simulink model "module_dynamic_merge_2018b"  (R2018b)
settings: Solver=FixedStepAuto  StartTime=0.0  StopTime=inf  FixedStep=0.001  RelTol=1e-3
settings Model: DataDictionary=LCplanning.sldd  Creator=lenovo  LastModifiedBy=lenovo
settings DataIOCC: ReturnWorkspaceOutputs=on

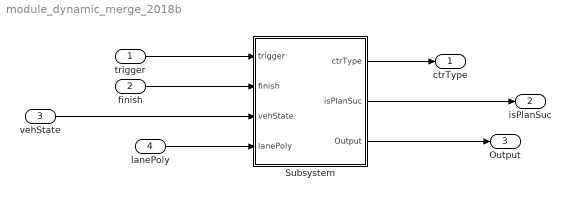
== system module_dynamic_merge_2018b ==
  trigger : Inport
  finish : Inport  Port=2
  vehState : Inport  Port=3  OutDataTypeStr=Bus: vehStates
  "lanePoly " : Inport  Port=4  OutDataTypeStr=Bus: lanePoly
  Subsystem : Subsystem
  ctrType : Outport  OutDataTypeStr=double
  isPlanSuc : Outport  Port=2  OutDataTypeStr=int8
  Output : Outport  Port=3  OutDataTypeStr=Bus: PlanningOutput
  wires:
  trigger/1 -> Subsystem/1(trigger)
  finish/1 -> Subsystem/2(finish)
  vehState/1 -> Subsystem/3(vehState)
  "lanePoly "/1 -> Subsystem/4("lanePoly ")
  Subsystem/1(ctrType) -> ctrType/1
  Subsystem/2(isPlanSuc) -> isPlanSuc/1
  Subsystem/3(Output) -> Output/1

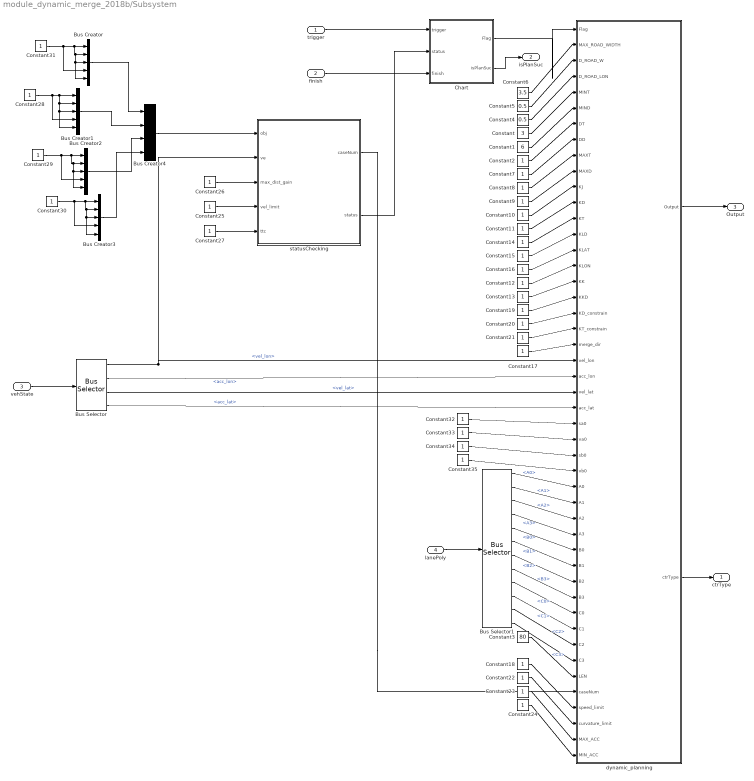
== system module_dynamic_merge_2018b/Subsystem ==
  trigger : Inport
  finish : Inport  Port=2
  vehState : Inport  Port=3  OutDataTypeStr=Bus: vehStates
  "lanePoly " : Inport  Port=4  OutDataTypeStr=Bus: lanePoly
  Bus Creator{,1..3} (4 alike) : BusCreator  Inputs=5  OutDataTypeStr=Bus: ObjInfo
  Bus Creator4 : BusCreator  Inputs=4  OutDataTypeStr=Bus: SelectedObject
  Bus Selector : BusSelector  OutputSignals=vel_lon,acc_lon,vel_lat,acc_lat
  Bus Selector1 : BusSelector  OutputSignals=A0,A1,A2,A3,B0,B1,B2,B3,C0,C1,C2,C3
  Chart : Stateflow chart  TreatAsAtomicUnit=on
  Constant : Constant  Value=3
  Constant1 : Constant  Value=6
  Constant{2,7..35} (30 alike) : Constant
  Constant3 : Constant  Value=80  OutDataTypeStr=double
  Constant4 : Constant  Value=0.5
  Constant5 : Constant  Value=0.5
  Constant6 : Constant  Value=3.5
  dynamic_planning : MATLAB Function  TreatAsAtomicUnit=on
  statusChecking : MATLAB Function  TreatAsAtomicUnit=on
  ctrType : Outport  OutDataTypeStr=double
  isPlanSuc : Outport  Port=2  OutDataTypeStr=int8
  Output : Outport  Port=3  OutDataTypeStr=Bus: PlanningOutput
  wires:
  Constant2/1 -> dynamic_planning/7(DT)
  Constant5/1 -> dynamic_planning/3(D_ROAD_W)
  Bus Selector1/10 -> dynamic_planning/39(C1)  "<C1>"
  Constant19/1 -> dynamic_planning/18(KKD)
  Bus Creator4/1 -> statusChecking/1(obj)
  trigger/1 -> Chart/1(trigger)
  Constant/1 -> dynamic_planning/5(MINT)
  statusChecking/1(caseNum) -> dynamic_planning/43(caseNum)
  Bus Selector1/5 -> dynamic_planning/34(B0)  "<B0>"
  statusChecking/2(status) -> Chart/2(status)
  Constant11/1 -> dynamic_planning/12(KD)
  Constant34/1 -> dynamic_planning/28(sb0)
  Constant14/1 -> dynamic_planning/13(KT)
  Constant10/1 -> dynamic_planning/11(KJ)
  Chart/1(Flag) -> dynamic_planning/1(Flag)
  Bus Creator/1 -> Bus Creator4/1
  Bus Creator3/1 -> Bus Creator4/4
  Constant4/1 -> dynamic_planning/4(D_ROAD_LON)
  Constant27/1 -> statusChecking/5(ttc)
  Constant15/1 -> dynamic_planning/14(KLD)
  Constant33/1 -> dynamic_planning/27(va0)
  "lanePoly "/1 -> Bus Selector1/1
  Bus Selector/3 -> dynamic_planning/24(vel_lat)  "<vel_lat>"
  Bus Selector1/2 -> dynamic_planning/31(A1)  "<A1>"
  Bus Selector1/7 -> dynamic_planning/36(B2)  "<B2>"
  Constant16/1 -> dynamic_planning/15(KLAT)
  Constant1/1 -> dynamic_planning/6(MIND)
  Bus Creator2/1 -> Bus Creator4/3
  Constant17/1 -> dynamic_planning/21(merge_dir)
  finish/1 -> Chart/3(finish)
  Bus Selector1/12 -> dynamic_planning/41(C3)  "<C3>"
  Constant13/1 -> dynamic_planning/17(KK)
  Constant3/1 -> dynamic_planning/42(LEN)
  Constant30/1 -> Bus Creator3/4, Bus Creator3/3, Bus Creator3/5, Bus Creator3/2, Bus Creator3/1
  Constant31/1 -> Bus Creator/4, Bus Creator/3, Bus Creator/5, Bus Creator/2, Bus Creator/1
  Constant12/1 -> dynamic_planning/16(KLON)
  Bus Selector1/11 -> dynamic_planning/40(C2)  "<C2>"
  Bus Selector/1 -> statusChecking/2(ve), dynamic_planning/22(vel_lon)  "<vel_lon>"
  Constant20/1 -> dynamic_planning/19(KD_constrain)
  Bus Selector/4 -> dynamic_planning/25(acc_lat)  "<acc_lat>"
  Constant6/1 -> dynamic_planning/2(MAX_ROAD_WIDTH)
  dynamic_planning/2(ctrType) -> ctrType/1
  Chart/2(isPlanSuc) -> isPlanSuc/1
  Constant9/1 -> dynamic_planning/10(MAXD)
  Constant29/1 -> Bus Creator2/4, Bus Creator2/3, Bus Creator2/5, Bus Creator2/2, Bus Creator2/1
  vehState/1 -> Bus Selector/1
  Bus Selector1/9 -> dynamic_planning/38(C0)  "<C0>"
  dynamic_planning/1(Output) -> Output/1
  Constant22/1 -> dynamic_planning/45(curvature_limit)
  Constant28/1 -> Bus Creator1/4, Bus Creator1/1, Bus Creator1/2, Bus Creator1/3, Bus Creator1/5
  Constant7/1 -> dynamic_planning/8(DD)
  Constant25/1 -> statusChecking/4(vel_limit)
  Constant23/1 -> dynamic_planning/46(MAX_ACC)
  Constant24/1 -> dynamic_planning/47(MIN_ACC)
  Constant26/1 -> statusChecking/3(max_dist_gain)
  Bus Selector1/4 -> dynamic_planning/33(A3)  "<A3>"
  Constant21/1 -> dynamic_planning/20(KT_constrain)
  Constant8/1 -> dynamic_planning/9(MAXT)
  Bus Selector/2 -> dynamic_planning/23(acc_lon)  "<acc_lon>"
  Bus Creator1/1 -> Bus Creator4/2
  Bus Selector1/1 -> dynamic_planning/30(A0)  "<A0>"
  Constant35/1 -> dynamic_planning/29(vb0)
  Constant18/1 -> dynamic_planning/44(speed_limit)
  Bus Selector1/8 -> dynamic_planning/37(B3)  "<B3>"
  Bus Selector1/3 -> dynamic_planning/32(A2)  "<A2>"
  Bus Selector1/6 -> dynamic_planning/35(B1)  "<B1>"
  Constant32/1 -> dynamic_planning/26(sa0)

== matlab function module_dynamic_merge_2018b/Subsystem/dynamic_planning ==
  data: Flag input; MAX_ROAD_WIDTH input; Output output Bus: PlanningOutput; D_ROAD_W input; D_ROAD_LON input; MINT input; MIND input; DT input; DD input; MAXT input; MAXD input; KJ input; KD input; KT input; KLD input; KLAT input; KLON input; KK input; KKD input; KD_constrain input; KT_constrain input; merge_dir input; vel_lon input; acc_lon input; vel_lat input; acc_lat input; sa0 input; va0 input; sb0 input; vb0 input; A0 input; A1 input; A2 input; A3 input; B0 input; B1 input; B2 input; B3 input; C0 input; C1 input; C2 input; C3 input; LEN input; caseNum input; speed_limit input; curvature_limit input; MAX_ACC input; MIN_ACC input; ctrType output double
%% /****************************************************************************
% *  Automatic Lane Changing                                                   *
% *  Copyright (C) 2020 Yuncheng JIANG  yjiangbw@connect.ust.hk.               *
% *                                                                            *
% *  This file is part of Lane Changing functionals.                           *
% *                                                                            *
% *  This program is free software; you can redistribute it and/or modify      *
% *  it under the terms of the GNU General Public License version 3 as         *
% *  published by the Free Software Foundation.                                *
% *                                                                            *
% *  You should have received a copy of the GNU General Public License         *
% *  along with OST. If not, see <http://www.gnu.org/licenses/>.               *
% *                                                                            *
% *  Unless required by applicable law or agreed to in writing, software       *
% *  distributed under the License is distributed on an "AS IS" BASIS,         *
% *  WITHOUT WARRANTIES OR CONDITIONS OF ANY KIND, either express or implied.  *
% *  See the License for the specific language governing permissions and       *
% *  limitations under the License.                                            *
% *                                                                            *
% *  @file                                                                     *
% *  @brief                                                                    *
% *  Details.                                                                  *
% *                                                                            *
% *  @author   Yuncheng.JIANG                                                  *
% *  @email    yjiangbw@connect.ust.hk.                                        *
% *  @version  1.0.0.1( )                                                      *
% *  @date     /12/1/2020                                                      *
% *  @license  GNU General Public License (GPL)                                *
% *                                                                            *
% *----------------------------------------------------------------------------*
% *  Remark         : Description                                              *
% *----------------------------------------------------------------------------*
% *  Change History :                                                          *
% *  <Date>     | <Version> | <Author>       | <Description>                   *
% *----------------------------------------------------------------------------*
% *  2020/12/01 | 1.0.0.1   | Yuncheng.JIANG       | Create file               *
% *----------------------------------------------------------------------------*
% *                                                                            *
% *****************************************************************************/

%% following is the parameter value reference

% global MAX_ROAD_WIDTH D_ROAD_W D_ROAD_LON MINT MIND DT DD MAXT MAXD KJ KD KT KLD KLAT KLON KK KKD KD_constrain KT_constrain;
% global merge_dir lat_offset vel_lon acc_lon vel_lat acc_lat ; 
% global sa0 va0 sb0 vb0 
% global A0 A1 A2 A3 B0 B1 B2 B3
% global LEN caseNum
% global speed_limit curvature_limit MAX_ACC MIN_ACC
% 
% MAX_ROAD_WIDTH = 3 ; %  [m]
% D_ROAD_W = 0.5 ; %  [m]
% D_ROAD_LON = 0.5;
% DT = 1 ; % Delta T [s]
% MAXT = 6;% [s]
% MINT = 3; % [s]
% DD = 1 ; % Delta T [s]
% MAXD = 80;% [s]
% MIND = 40; % [s]
% KJ = 0.1;
% KT = 0.1;
% KD = 1;
% KLD = 1;
% KLAT = 1;
% KLON = 1;
% KK = 1;
% KKD = 1;
% KD_constrain = 0.1;
% KT_constrain = 1;
% 
% merge_dir = 1;
% vel_lon = 10;
% acc_lon = 0;
% vel_lat = 0;
% acc_lat = 0;
% lat_offset = -6;
% 
% sa0 = 0;
% va0 = 10;
% sb0 = 15;
% vb0 = 10; 
% 
% A0 = -3; A1 = -0.1; A2 = -0.001; A3 = -0.0001;
% B0 = 3; B1 = -0.1; B2 = -0.001; B3 = -0.00008;
% % we also have C parameters here
% 
% LEN = 80;
% caseNum = 2;
% speed_limit = 33.3; % which is 120kph;
% curvature_limit = 1/50;
% MAX_ACC = 4;
% MIN_ACC = -4;


%% the test declare that when caseNum == 4, it is a free lane changing.
% when caseNum != 4, it is merging lane changing.


%%
% frenet_data = check_status(cost_graph);
% cost_total = frenet_data(1);
% Te = frenet_data(2);
% de = frenet_data(3);
% se = frenet_data(4);
% [y_of_x,p_of_v,p_of_a] = conbination(frenet_data);
% toc; 
% 
% fprintf("the calculation time = %f  ms \r",1000*toc);
% 
% figure
% plot(p_of_v(:,1),p_of_v(:,2));
% title("y of x");
% figure
% plot(p_of_v(:,1),p_of_v(:,3));
% title("p of v");
% figure
% plot(p_of_a(:,1),p_of_a(:,3));
% title("p of a");

%%
function [Output,ctrType]  = dynamic_planning(Flag, MAX_ROAD_WIDTH, D_ROAD_W, D_ROAD_LON,...
    MINT, MIND, DT, DD, MAXT, MAXD, KJ, KD, KT, KLD, KLAT, KLON, KK, KKD, KD_constrain, KT_constrain,...
    merge_dir, vel_lon, acc_lon, vel_lat, acc_lat,...
    sa0, va0, sb0, vb0 ,A0, A1, A2, A3, B0, B1, B2, B3, C0, C1, C2, C3,LEN, caseNum,...
    speed_limit, curvature_limit, MAX_ACC, MIN_ACC)
    %% this function discrriminate two different sampling methods.
    % if caseNum ==4, it means this is simple lane changing, we change lane
    % without considering of velocity planning
    % if caseNum != 4, it means this is merging lane changing, we apply
    % x(t)-y(t) method to plan spatially and temporally. 
    
%     global Flag MAX_ROAD_WIDTH D_ROAD_W D_ROAD_LON MINT MIND DT DD MAXT MAXD KJ KD KT KLD KLAT KLON KK KKD KD_constrain KT_constrain;
%     global merge_dir lat_offset vel_lon acc_lon vel_lat acc_lat ;
%     global sa0 va0 sb0 vb0 
%     global A0 A1 A2 A3 B0 B1 B2 B3
%     global LEN caseNum
%     global speed_limit curvature_limit MAX_ACC MIN_ACC Flag
    
    if Flag == 3
        [reference] = reference_line_generator(A0,A1,A2,A3, B0,B1,B2,B3, LEN);
    else 
        [reference] = reference_line_generator(A0,A1,A2,A3, C0,C1,C2,C3, LEN);
    end
    
    ctrType = 0;
    
    if Flag == 0
        output = zeros(500,8);
        Output = transition_to_BUS(output);
        ctrType = 0; 
        
    elseif Flag == 1
        output = ones(500,8);
        output(:,7) = 2;
      Output = transition_to_BUS(output);
        ctrType = 2;
    else
        if caseNum == 4 || caseNum == 2
            % Case4 does simplified lane changing, while Case2 does lane
            % changing without front vehicles
            [cost_graph] = calc_frenet_paths_free(Flag, MAX_ROAD_WIDTH, D_ROAD_W, D_ROAD_LON,...
                MINT, MIND, DT, DD, MAXT, MAXD, KJ, KD, KT, KLD, KLAT, KLON, KK, KKD, KD_constrain, KT_constrain,...
                merge_dir, vel_lon, acc_lon, vel_lat, acc_lat,...
                sa0, va0, sb0, vb0 ,A0, A1, A2, A3, B0, B1, B2, B3, C0, C1, C2, C3,LEN, caseNum,...
                speed_limit, curvature_limit, MAX_ACC, MIN_ACC);

            D0 = 1/2*(A0 + B0); % how to determine D0 is still a problem??? calculate using correct 1/2*(A0 + B0)??
            Ti = cost_graph(1,2);
            Di =cost_graph(1,3);
            [ref_bezier] = ref_bezier_generation(reference, D0,Ti,Di);
            trajs_new_origin = reference_generation(reference, ref_bezier);% 

            delta_heading_rad = calculat_delta_heading(reference, trajs_new_origin);
            delta_heading_deg = rad_to_deg(delta_heading_rad); % If you need 
            kappa = calculate_kappa_oneshot(trajs_new_origin);
            adding = zeros(length(kappa),2)-1;
            output = [trajs_new_origin,ref_bezier,delta_heading_rad,kappa,adding];
            ctrType = 1;
            Output = transition_to_BUS(output);
            
            
%             the output contains infomation as follow: 
%             1,2 cols: under vehicle coordinate, the x,y positions of planned
%             trajectories;
%             3,4 cols: w.r.t longitudinal intergration s, the lateral offset on
%             each sampled s, offset to left of reference line is positive, and
%             the other side is negative;
%             5 cols: delta_heading of matched point vectors between reference
%             line and planned trajs, anti-clock wise from reference to planned
%             trajs is positive;
%             6 cols: planned trajs kappa, vehicle turing left is positive and
%             turning right is negative;
%             7 cols: velocity profile along the planned trajectory.
%             8 cols: acceleration profile along the planned trajectory.
        else
            % do merging method lane changing
            output = [];
            [cost_graph] = calc_frenet_paths_constraint(Flag, MAX_ROAD_WIDTH, D_ROAD_W, D_ROAD_LON,...
                MINT, MIND, DT, DD, MAXT, MAXD, KJ, KD, KT, KLD, KLAT, KLON, KK, KKD, KD_constrain, KT_constrain,...
                merge_dir, vel_lon, acc_lon, vel_lat, acc_lat,...
                sa0, va0, sb0, vb0 ,A0, A1, A2, A3, B0, B1, B2, B3, C0, C1, C2, C3,LEN, caseNum,...
                speed_limit, curvature_limit, MAX_ACC, MIN_ACC);
            
            cost_graph_optimal = check_status(cost_graph,speed_limit, curvature_limit, MAX_ACC, MIN_ACC);
            
            [y_of_x,p_of_v,p_of_a] = conbination(cost_graph_optimal);
            
            [ref_poly] = ref_poly_generation(reference, y_of_x);
            trajs_new_origin = reference_generation(reference, ref_poly);% 
            [v_profile] = velocity_intepolation(p_of_v,reference);
            [a_profile] = acc_intepolation(p_of_a,reference);
            delta_heading_rad = calculat_delta_heading(reference, trajs_new_origin);
            delta_heading_deg = rad_to_deg(delta_heading_rad); % If you need 
            kappa = calculate_kappa_oneshot(trajs_new_origin);
            output = [trajs_new_origin,ref_poly,delta_heading_rad,kappa,v_profile,a_profile];
            ctrType = 3;
            Output = transition_to_BUS(output);
        end
    end
end

%%
function [ref_bezier] = ref_bezier_generation(reference_1, D0, Ti, Di)
%% this function generate bezier curve information 
% input: the centerline reference_1, bezier curve control points
% output: the matrix is in dimension of n by 2, with its first col
% longitudinal integration length, second col lateral offset with respect
% to center line.
% notice: shifting to left is positive, and vice versa. 
S = 0;
    ref_bezier = [[],[]];
    index =1;
    while S < Ti && (index+1) <= length(reference_1)
        p = Bezierfrenet_5(D0, Ti, Di,S);
        ref_bezier =[ref_bezier; p];
        S = S + sqrt((reference_1(index+1,1)-reference_1(index,1))^2 + ...
            (reference_1(index+1,2)-reference_1(index,2))^2);
        index = index + 1;
    end
end

%%
function [v_profile] = velocity_intepolation(p_of_v,reference)
    
    if isempty(p_of_v) 
        fprintf("error in optimal p_of_v.");
        v_profile = [];
        return;
    end
    
    if isempty(reference)  
        fprintf("error in optimal reference.");
        v_profile = [];
        return;
    end
    
    S = 0;
    v_profile = [];
    index =1;
    X = p_of_v(:,1);
    V = p_of_v(:,3);
    XMAX = min(reference(end,1),X(end));
    
    while S <= XMAX && (index+1) <= length(reference)
        
        v = [S,interp1(X,V,S,'spline')];
        
        v_profile =[v_profile; v];
        S = S + sqrt((reference(index+1,1)-reference(index,1))^2 + ...
            (reference(index+1,2)-reference(index,2))^2);
        index = index + 1;
    end


end


function [a_profile] = acc_intepolation(p_of_a,reference)
    
    if isempty(p_of_a) 
        fprintf("error in optimal p_of_a.");
        a_profile = [];
        return;
    end
    
    if isempty(reference)  
        fprintf("error in optimal reference.");
        a_profile = [];
        return;
    end
    
    S = 0;
    a_profile = [];
    index =1;
    X = p_of_a(:,1);
    A = p_of_a(:,3);
    XMAX = min(reference(end,1),X(end));
    
    while S <= XMAX && (index+1) <= length(reference)
        
        a = [S,interp1(X,A,S,'spline')];
        
        a_profile =[a_profile; a];
        S = S + sqrt((reference(index+1,1)-reference(index,1))^2 + ...
            (reference(index+1,2)-reference(index,2))^2);
        index = index + 1;
    end



end
%%
function [ref_poly] = ref_poly_generation(reference, y_of_x)
%% this function generate polynomial curve informaion
    if isempty(y_of_x)
        fprintf("error in optimal y_of_x.");
        ref_poly = [];
        return;
    end
    
    S = 0;
    ref_poly = [[],[]];
    index =1;
    X = y_of_x(:,1);
    Y = y_of_x(:,2);
    XMAX = min(reference(end,1),X(end));
    
    while S <= XMAX && (index+1) <= length(reference)
        
        p = [S,interp1(X,Y,S,'spline')];
        
        ref_poly =[ref_poly; p];
        S = S + sqrt((reference(index+1,1)-reference(index,1))^2 + ...
            (reference(index+1,2)-reference(index,2))^2);
        index = index + 1;
    end
end





%%
function [y_of_x,p_of_v,p_of_a] = conbination(frenet_data)
    if isempty(frenet_data)
        y_of_x = [ ];
        p_of_v = [ ];
        p_of_a = [ ];
        fprintf("error in optimal cost graph.");
        return;
    end
    Te = frenet_data(2); 
    a = zeros(6,1);
    b = zeros(6,1);
    for i = 5:10
        a(i-4) = frenet_data(i);
        b(i-4) = frenet_data(i+6);
    end
    
    xt = [];
    yt = [];
    vxt = [];
    vyt = [];
    axt = [];
    ayt = [];
    
    for t = 0:0.05:Te
        a0 = a(1); a1 = a(2); a2 = a(3); a3 = a(4);
        a4 = a(5); a5 = a(6); b0 = b(1); b1 = b(2);
        b2 = b(3); b3 = b(4); b4 = b(5); b5 = b(6);
        [yt] = [yt,calc_point(a0,a1,a2,a3,a4,a5,t)];
        [vyt] = [vyt, calc_first_derivative(a1,a2,a3,a4,a5,t)];
        [ayt] = [ayt, calc_second_derivative(a2,a3,a4,a5,t)];
        [xt] = [xt, calc_point(b0,b1,b2,b3,b4,b5,t)];
        [vxt] =[ vxt, calc_first_derivative(b1,b2,b3,b4,b5,t)];
        [axt] = [axt, calc_second_derivative(b2,b3,b4,b5,t)];
    end
    
    velocity = sqrt(vxt.^2 + vyt.^2);
    acceleration = sign(axt) .* sqrt(axt.^2 + ayt.^2);
    y_of_x = [xt',yt'];
    p_of_v = [xt',yt',velocity'];
    p_of_a = [xt',yt',acceleration'];
        
end

%%
function cost_graph_optimal = check_status(cost_graph,speed_limit, curvature_limit, MAX_ACC, MIN_ACC)

%     global MAX_ROAD_WIDTH D_ROAD_W D_ROAD_LON MINT MIND DT DD MAXT MAXD KJ KD KT KLD KLAT KLON KK KKD KD_constrain KT_constrain;
%     global merge_dir lat_offset vel_lon acc_lon vel_lat acc_lat ;
%     global sa0 va0 sb0 vb0 
%     global A0 A1 A2 A3 B0 B1 B2 B3
%     global LEN caseNum
%     global speed_limit curvature_limit MAX_ACC MIN_ACC   
    
    i = 1;
    COND = 1;
    if isempty(cost_graph)
        cost_graph_optimal=  [];
        fprintf("error in cost graph.");
        return;
    end
    
    cost_graph_optimal = cost_graph(1,:);
    while COND == 1
        frenet_data = cost_graph(i,:);
        Te = frenet_data(2);  
        a = zeros(1,6);
        b = zeros(1,6);
        for i = 5:10
            a(i-4) = frenet_data(i);
            b(i-4) = frenet_data(i+6);
        end
    
        xt = [];
        yt = [];
        vxt = [];
        vyt = [];
        axt = [];
        ayt = [];

        for t = 0:0.1:Te
            a0 = a(1); a1 = a(2); a2 = a(3); a3 = a(4);
            a4 = a(5); a5 = a(6); b0 = b(1); b1 = b(2);
            b2 = b(3); b3 = b(4); b4 = b(5); b5 = b(6);
            [yt] = [yt,calc_point(a0,a1,a2,a3,a4,a5,t)];
            [vyt] = [vyt, calc_first_derivative(a1,a2,a3,a4,a5,t)];
            [ayt] = [ayt, calc_second_derivative(a2,a3,a4,a5,t)];
            [xt] = [xt, calc_point(b0,b1,b2,b3,b4,b5,t)];
            [vxt] =[ vxt, calc_first_derivative(b1,b2,b3,b4,b5,t)];
            [axt] = [axt, calc_second_derivative(b2,b3,b4,b5,t)];
        end
        
        trajs = [xt',yt'];
        velocity = sqrt(vxt.^2 + vyt.^2);
        acceleration = sign(axt) .* sqrt(axt.^2 + ayt.^2);
        kappa = calculate_kappa_oneshot(trajs);
        
        if ((max(abs(velocity))<= speed_limit) && (max(acceleration)<=MAX_ACC)...
                && (min(acceleration) >= MIN_ACC) && (max(abs(kappa)) < curvature_limit))
            cost_graph_optimal = cost_graph(i,:);
            COND = 2;
        end
        
        i = i+1;
        
        if  i > size(cost_graph,1)
            COND = 2;
            cost_graph_optimal = cost_graph(1,:);
        end
    end
        
        
end
%%
function [cost_graph] = calc_frenet_paths_constraint(Flag, MAX_ROAD_WIDTH, D_ROAD_W, D_ROAD_LON,...
    MINT, MIND, DT, DD, MAXT, MAXD, KJ, KD, KT, KLD, KLAT, KLON, KK, KKD, KD_constrain, KT_constrain,...
    merge_dir, vel_lon, acc_lon, vel_lat, acc_lat,...
    sa0, va0, sb0, vb0 ,A0, A1, A2, A3, B0, B1, B2, B3, C0, C1, C2, C3,LEN, caseNum,...
    speed_limit, curvature_limit, MAX_ACC, MIN_ACC)

% @breif this is the function to sample all possible candidate in cases of
    % constrained merging scenarios. it uses x(t)-y(t) method, which means it
    % outputs spatial and temporal profiles.

% input: 
    % directly call all global data
    
% output:
    % cost graph maintains all sampled candidate information, which is as
    % follow: The first col is the total cost. The second col is Ti, which
    % is time T. The third col is di, which is terminal lateral offset. The
    % fourth col is si, which is terminal longitudinal distance.
    
    
%     global MAX_ROAD_WIDTH D_ROAD_W D_ROAD_LON MINT MIND DT DD MAXT MAXD KJ KD KT KLD KLAT KLON KK KKD KD_constrain KT_constrain;
%     global merge_dir lat_offset vel_lon acc_lon vel_lat acc_lat ;
%     global sa0 va0 sb0 vb0 
%     global A0 A1 A2 A3 B0 B1 B2 B3
%     global LEN caseNum
%     global speed_limit curvature_limit MAX_ACC MIN_ACC
    
    frenet_paths =[]; % initiate it with empty
    cost_graph = []; % initiate it with empty
    
    if merge_dir == 1 % merging to left lane
        lower_bound = -MAX_ROAD_WIDTH / 2;
        upper_bound = 0;
    else % merging to right lane
        lower_bound = 0;
        upper_bound = MAX_ROAD_WIDTH / 2;
    end
    
    for Ti = MINT : DT : MAXT
        for di = lower_bound : D_ROAD_W : upper_bound
            xs = 1/2*(A0 + B0); % how to determine D0 is still a problem??? calculate using correct 1/2*(A0 + B0)??
            vxs = vel_lat;
            axs = acc_lat;
            %Ti is sampling on T
            xe = di; % sampling on lateral offset
            vxe = 0;
            axe = 0;
            [a0, a1, a2, a3, a4,a5] = quintic_polynomial(xs, ...
                vxs, axs, xe, vxe, axe,Ti);
            [jerk_bar_lat] = cal_j_bar(a3,a4,a5,Ti);
            [d_bar_lat] = calc_d_bar(a0,a1,a2,a3,a4,a5,Ti);
            cost_total_lat = KJ * jerk_bar_lat + KD_constrain * d_bar_lat + KT_constrain * Ti;
            
            
            xs = 0;
            vxs = vel_lon;
            axs = acc_lon;

            [xe,sa,sb] = cal_xe(caseNum, sa0,sb0,va0,vb0,Ti); % go to function definition for details
            
            delta_s = 1/4 * (sb - sa); % how to determine ??? we still have not make sure 
            
            vxe = 1/2 * (va0 + vb0);
            axe = 0;
            
            for si = xe - delta_s : D_ROAD_LON : xe + delta_s
           
                [b0, b1, b2, b3, b4, b5] = quintic_polynomial(xs, ...
                    vxs, axs, xe, vxe, axe,Ti);
                [jerk_bar_lon] = cal_j_bar(b3,b4,b5,Ti);
                delta_d = abs(si - xe);

                cost_total_lon = KJ * jerk_bar_lon + KLD * delta_d + KT_constrain * Ti;
               
                cost_total = KLAT * cost_total_lat + KLON * cost_total_lon;
                cost_graph = [cost_graph;[cost_total, Ti, di, si,...
                    a0, a1, a2, a3, a4, a5, b0, b1, b2, b3, b4, b5]];
            end
        end
    end
    cost_graph = sortrows(cost_graph);
end

%%
function [cost_graph] = calc_frenet_paths_free(Flag, MAX_ROAD_WIDTH, D_ROAD_W, D_ROAD_LON,...
    MINT, MIND, DT, DD, MAXT, MAXD, KJ, KD, KT, KLD, KLAT, KLON, KK, KKD, KD_constrain, KT_constrain,...
    merge_dir, lat_offset, vel_lon, acc_lon, vel_lat, acc_lat,...
    sa0, va0, sb0, vb0 ,A0, A1, A2, A3, B0, B1, B2, B3, C0, C1, C2, C3,LEN, caseNum,...
    speed_limit, curvature_limit, MAX_ACC, MIN_ACC)

%     global MAX_ROAD_WIDTH D_ROAD_W D_ROAD_LON MINT MIND DT DD MAXT MAXD KJ KD KT KLD KLAT KLON KK KKD;
%     global merge_dir lat_offset vel_lon acc_lon vel_lat acc_lat ;
%     global sa0 va0 sb0 vb0 
%     global A0 A1 A2 A3 B0 B1 B2 B3
%     global LEN caseNum
%     global speed_limit
% lateral_offset, MAX_ROAD_WIDTH,...
    %D_ROAD_W, MINT,DT,MAXT,KJ,KD,KT,KK,KKD
    
% KJ is the cost weight of the jerk;
% KD is the cost weight of lateral offset with respect to the reference
% line;
% KT is the cost weight of the longitudinal distance 
% KK is the cost weight of curvature
% KKD is the cost weight of the derivative of curvature
% KO is the cost weight of ostacle distance

    D0 = lat_offset; % 0.5 * (a0 + b0) is also lateral_offset in lane keeping system;
    frenet_paths = [];
    cost_graph = []; 
    % we store all candicates' cost info in this matrix for review,
    % but remember that it is not necessary when the parameters are well turned.
    if merge_dir == 1 % merging to left lane
        lower_bound = -MAX_ROAD_WIDTH / 2;
        upper_bound = 0;
    else % merging to right lane
        lower_bound = 0;
        upper_bound = MAX_ROAD_WIDTH / 2;
    end
    
    j = 1;
    for di = lower_bound : D_ROAD_W : upper_bound
        for Ti =  MIND: DD: MAXD
            p = [];
            for t = 0:0.1:Ti
                p = [p; Bezierfrenet_3(D0, Ti, di,t)];
            end
            
            [pd] = calculate_pd(p);
            [pdd] = calculate_pdd(p);
            [k] = calculate_kappa(p,pd,pdd);
            [kappa_d] = calculate_kappa_d(p,k);
           
            cost_J = mean(abs(pdd));
            cost_D = mean(abs(p(:,2)));
            cost_T = Ti;
            cost_K = mean(abs(k));
            cost_KD = mean(abs(kappa_d));
                    
            cost_total = KJ * cost_J + KD * cost_D + cost_T * KT +...
                cost_K* KK + KKD * cost_KD;
            cost_graph = [cost_graph;[cost_total,Ti,di,cost_J,cost_D,cost_T,cost_K,cost_KD]];
            
%         cost_T = regularization(cost_T);
%         cost_D = regularization(cost_D);

        end
    end
        cost_graph = sortrows(cost_graph); % important info is in the first 3 columns: tatal_cost. Ti, di;
end


%%



function [a0, a1, a2, a3, a4,a5] = quintic_polynomial(xs, ...
    vxs, axs, xe, vxe, axe,T)
% A = [0,0,0,0,0,1; T^5,T^4,T^3,T^2,T,1;...
%     0,0,0,0,1,0 ; 5*T^4  4*T^3 3*T^2 2*T 1 0 ; ...
%     0 0 0 2 0 0; 20*T^3 12*T^2 6*T 2 0 0];
% b = [xs, xe, vxs, vxe, axs, 0]';
% x = A\b;
% a5 = x(1);
% a4 = x(2);
% a3 = x(3);
% a2 = x(4);
% a1 = x(5);
% a0 = x(6);
A = [T^3 T^4 T^5; 3*T^2 4*T^3 5*T^4; 6*T 12*T^2 20*T^3];
b = [(xe - xs  - vxs*T - 0.5*axs*T^2); (vxe- vxs - axs*T ); (axe - axs)];

if det(A) == 0
    a0 = [];
    a1 = [];
    a2 = [];

    a3 = [];
    a4 = [];
    a5 = [];  
    
    fprintf('cannot calculate quintic polynomial paras.');
    return;
end
    
    
x = A\b;
a0 = xs;
a1 = vxs;
a2 = axs/2;

a3 = x(1);
a4 = x(2);
a5 = x(3);
end

function [xt] = calc_point(a0,a1,a2,a3,a4,a5,t)
xt = a0 + a1 * t + a2 * t ^2 + a3 * t^3 + a4 * t^4 + a5 * t^5;
end

function [d_bar] = calc_d_bar(a0,a1,a2,a3,a4,a5,T)
    xt = [];
    for t =0 : 0.1 : T
        xt = [xt, calc_point(a0,a1,a2,a3,a4,a5,t)];
    end
    d_bar = mean(abs(xt));
end

function [jerk_bar] = cal_j_bar(a3,a4,a5,T)
    jt = [];
    for t =0 : 0.1 : T
        jt = [jt, calc_third_derivative(a3,a4, a5,t)];
    end
    jerk_bar = mean(abs(jt));
end

function [xe,sa,sb] = cal_xe(caseNum, sa0,sb0,va0,vb0,Ti)
    CONST =60; % It remains uncertain how how to choose a properiate distance CONST.    
    switch caseNum
        case 1 % in this case, we have vehicle a and vehilce b;
            sa = sa0 + va0 * Ti; % a_vehicle: the nearest adjacent vehicle which is declared as rear vehicle;
            sb = sb0 + vb0 * Ti; % b_vehilce: the nearest adjacent vehicle that is in front of the a_vehicle(front vehicle);
            xe = sa + (sb - sa) * 2/3;% 1/2 * (sb + sa);
        case 2 % in this case, we have only vehicle a;
           sa = sa0 + va0 * Ti;
           sb = sa + CONST; % the distance between two vehicles is CONST
           xe = sa + (sb - sa) * 2/3;% 1/2 * (sb + sa);
        otherwise % in this case, we only have vehicle b;
           sb = sb0 + vb0 * Ti;
           sa =  sb - CONST; % the distance between two vehicles is CONST
           xe = sa + (sb - sa) * 2/3;% 1/2 * (sb + sa);
    end              
end


%%  
function [reference] = reference_line_generator(a0,a1,a2,a3, b0,b1,b2,b3, LEN)
%% in this function, we use the left and right lane polynomials to generate
% a reference center line
% input: left lane polynomials, right lane polynomials, LEN(length of reference)
% output: reference center line polynomials
reference = [[],[]];
if LEN == 0
    fprintf('LEN = 0, reference cannot be generated. \r')
    return;
end

for i = 0:0.2:LEN
    y = 0.5 * ( (a0 + a1 * i + a2 * i^2 + a3 * i^3) + (b0 + b1 * i + b2 * i^2 + b3 * i^3));
    reference =  [reference; [i,y]];
end
end
%%
function y = f_a(a0, a1, a2, a3, x)
%% calculate polynomial y values
    y = a0 + a1 * x + a2 * x^2 + a3 * x^3;
end

function y = f_b(b0, b1, b2, b3, x)
%% calculate polynomial y values
    y = b0 + b1 * x + b2 * x^2 + b3 * x^3;
end

function y = deg_to_rad(x)
%% deg to rad unit switch
    y = x * pi / 180;
end

function y = rad_to_deg(x)
%% rad to degree unit switch
    y = x * 180 / pi;
end
%%
function [reference] = reference_line_generator_frenet(a0,a1,a2,a3, b0,b1,b2,b3, LEN)
%% this function generates center line in discrete form
% input: the left lane and right lane polynomials parameters, and
% longitudinal LEN(how long we want to generate such a curve)
% output: using frenet method to generate the ceterline position in x and
% y

if LEN == 0
    fprintf('LEN = 0, reference cannot be generated. \r');
    return;
end

S = 0;
iter = 0;
x_a = 0;
x_b = 0;

delta_x = 0.02;
RESOLUTION = 0.2;
y_a_pre = f_a(a0,a1,a2,a3, x_a);
y_b_pre = f_b(b0,b1,b2,b3, x_b);
reference = [x_a, 0.5*(y_a_pre + y_b_pre)];
while S < LEN

    s_a = 0;
    s_b = 0;
    while s_a < RESOLUTION
        x_a = x_a + delta_x;
        y_a = f_a(a0,a1,a2,a3, x_a);
        s_a = s_a + sqrt( delta_x^2 + (y_a - y_a_pre)^2);
        y_a_pre = y_a;
    end
    
    while s_b < RESOLUTION 
        x_b = x_b + delta_x;
        y_b = f_b(b0,b1,b2,b3, x_b);
        s_b = s_b + sqrt( delta_x^2 + (y_b - y_b_pre)^2);
        y_b_pre = y_b;
    end
    
    S = S + RESOLUTION;
    reference = [reference; [0.5*(x_a + x_b), 0.5*(y_a + y_b) ]];
    
    iter = iter + 1;
    if iter >= 5000
        print("while loop too long, missing error! \r")
        break;
    end
    
end
end


function [p] = Bezierfrenet_3(D0, Ti, Di,t)
    %% 
    % D0 initial lateral offset, which is current vehicle lateral offset with
    % respect to center line of current lane 
    % Ti:  the longitudinal position of the desired target
    % Di the lateral position of the desired target
    % t sampling step in discretization

    %set the four control point
    p0 = [0, D0];
    p1 = [Ti/2, D0];
    p2 = [Ti/2, Di];
    p3 = [Ti, Di];

    p = (1-(t)/Ti)^3*p0 + 3*(1-(t)/Ti)^2*(t)/Ti*p1 + ...
     3*(1-(t)/Ti)*((t)/Ti)^2*p2 + ((t)/Ti)^3*p3;
end

function [p] = Bezierfrenet_5(D0, Ti, Di,t)
%% this function provides the bezier curve information. 
% when given control points information, it can generate y values based on
% given x values.
    p0 = [ 0, D0];
    p1 = [0.25 * Ti, D0];
    p2= [0.5 *Ti, D0];
    p3 =[ 0.5 * Ti, Di];
    p4 =[ 0.75 * Ti, Di];
    p5 = [Ti, Di];
  %generate a fifth order bezier curve

    p= (1-(t)/Ti)^5*p0 + 5*(1-(t)/Ti)^4*((t)/Ti)*p1 + 10*(1-(t)/Ti)^3*((t)/Ti)^2*p2 +...
     10*(1-(t)/Ti)^2*((t)/Ti)^3*p3 +5*(1-(t)/Ti)*((t)/Ti)^4*p4 + ((t)/Ti)^5*p5;

end 
%%

function [trajs_new] = reference_generation(trajs_local, p_store)
%% this function provides method of generating changing lane discrete positions.    
% inputs: here the trajs_local is a vector<vector<double>>,with its dimension
%n by 2, the p_store store the information Bezier curve generaion
%function creates, which are longitudinal 's' and 'lateral offset', which
%is also in dimension of n by 2. 
%output: with the two inputs info, we are able to generate under vehicle
%coordinate the changing lane positions by doing position shift, based on
%the original trajs_local, in frenet direction with offset info provided by
%p_store.
if (isempty(trajs_local)) || (length(trajs_local) == 0)
    fprintf('reference trajs is not well generated! \r');
    trajs_new= [];
    return;
end

if isempty(p_store) || (length(p_store) == 0)
    fprintf('offset Bezier curve is not well generated! \r');
    trajs_new= [];
    return;
end

    trajs_new = [[ ],[ ]];
    for i = 1: min(length(p_store), length(trajs_local))
%         if (i + current_index) > length(waypoint)
%             break;
%         end
        d = p_store(i,2);
        if trajs_local(i,1) == 0
            theta = 0;
        else
            theta = atan(trajs_local(i,2) / trajs_local(i,1));
        end
        
        if (theta>-pi/2 && theta <=0)
            x = trajs_local(i,1) - d * sin(theta);
            y = trajs_local(i,2) + d * cos(theta);
            trajs_new = [trajs_new ; [x,y]];
        elseif (theta>0 && theta < pi/2)
            x = trajs_local(i,1) - d * sin(theta);
            y = trajs_local(i,2) + d * cos(theta);
            trajs_new = [trajs_new ; [x,y]];    
        else
           fprintf("it seems that the reference line is unacceptable!");
        end
    end
end

%%
function [k] = calculate_kappa(p,pd,pdd) 
    k = zeros(length(p),1);
    for i  = 1:length(p)
             k(i) = (pdd(i))/((1+pd(i)^2)^(1.5));
         end
    end

%%
function [pd] = calculate_pd(p)
    % calculate the first derivatives
    pd = zeros(length(p),1);
    for i = 1:length(p)-1
     pd(i) = (p(i+1,2)-p(i,2))/(p(i+1,1)-p(i,1));
    end
end

%%
function [pdd] = calculate_pdd(p)
    % calculate the second derivatives
     pdd = zeros(length(p),1);
     for i =2: length(p)-1
         pdd(i) = (p(i+1,2)-2*p(i,2) + p(i-1,2))/(0.5*(-p(i-1,1)+p(i+1,1)))^2;
    %    pdd(i) = (p(i+1,2)-2*p(i,2) + p(i-1,2))/(-p(i,1)+p(i+1,1))^2;
     end
end

%%
function [kappa_d] = calculate_kappa_d(p,k)
    kappa_d = zeros(length(p),1);
    kappa_d(1) = 0;
    for i = 2: length(p)
        kappa_d(i) = (k(i)-k(i-1))/norm(p(i,:)- p(i-1,:));
    end
end

%%
function [xt] =calc_first_derivative(a1,a2,a3,a4,a5,t)
xt = a1 + 2 * a2 * t + 3 * a3 * t^2 + 4 * a4 * t^3  +  5 * a5 * t^4;
end

%%
function [xt]  = calc_second_derivative(a2,a3,a4,a5,t)
xt = 2* a2 + 6* a3 * t + 12 * a4 * t^2 + 20* a5 *t^3;
end

%%
function [xt] = calc_third_derivative(a3,a4,a5,t)
xt =6 * a3 + 24 * a4 * t + a5 * t^2;
end

function [delta_heading] = calculat_delta_heading(center_line, traj_new)
    LEN = min(length(center_line), length(traj_new));
    delta_heading = [0];
    for i = 1: LEN-1
        x1 = center_line(i+1,1) - center_line(i,1);
        y1 = center_line(i+1,2) - center_line(i,2);
        x2 = traj_new(i+1,1) - traj_new(i,1);
        y2 = traj_new(i+1,2) - traj_new(i,2);
        delta_theta =  (x1 * x2 + y1 * y2) / (sqrt(x1^2 + y1^2) * sqrt(x2^2 + y2^2));
        delta_heading =  [delta_heading; acos(delta_theta)];
    end
end
%%

function [kappa] = calculate_kappa_oneshot(trajs_new)

% this function provide the method of generating a sequence of curvature(kappa) 
% input: a sequence of discrete points with position x and y.
% output: a sequence of kappa on each point.
% notice: vehicle turning right has negative curvature, and vice versa.

if (isempty(trajs_new)) || (length(trajs_new) == 0)
    fprintf('changing lane trajs is not well generated! \r');
    kappa = zeros(length(trajs_new),1);
    return;
end

    pd = zeros(length(trajs_new),1);
    pdd = zeros(length(trajs_new),1);
    kappa = zeros(length(trajs_new),1);
    
    % calculate the first derivatives
    
    for i = 1:length(trajs_new)-1
        
        if (trajs_new(i+1,1)-trajs_new(i,1)) == 0
            denominator_pd = 0.001;
        else
            denominator_pd = trajs_new(i+1,1)-trajs_new(i,1);
        end
        
        pd(i) = (trajs_new(i+1,2)-trajs_new(i,2))/denominator_pd;   
    end
    pd(length(trajs_new)) = pd(length(trajs_new)-1);
    % calculate the second derivatives
    pdd(1) = 0;
    for i =2: length(trajs_new)-1
        
        if (0.5*(-trajs_new(i-1,1) + trajs_new(i+1,1)))^2 == 0
            denominator_pdd = 0.001;
        else
            denominator_pdd = 0.5*(-trajs_new(i-1,1) + trajs_new(i+1,1))^2;
        end
        
        pdd(i) = (trajs_new(i+1,2)-2*trajs_new(i,2) +...
            trajs_new(i-1,2))/denominator_pdd;
    end
    pdd(length(trajs_new)) = pdd(length(trajs_new)-1);
    
    for i  = 1:length(trajs_new)
        kappa(i) = (pdd(i))/((1+pd(i)^2)^(1.5));
    end
end

function Output = transition_to_BUS(output)
%     
    size_of_out = length(output);
    
    
    if isempty(output)
        output = ones(500,8);
    elseif size(output,2) ~= 8
        output = ones(500,8);
    else
        if size_of_out < 500
            output = [output; zeros((500 - size_of_out),8)];
        else
            output = output(1:500,:);
        end
    end

%     output = ones(500,8);  
 
    Output.x = output(1:500,1);
    Output.y = output(1:500,2);
    Output.s = output(1:500,3);
    Output.lat_offset = output(1:500,4);
    Output.delta_theta = output(1:500,5);
    Output.kappa = output(1:500,6);
    Output.v_profile = output(1:500,7);
    Output.a_profile = output(1:500,8);
    
end

== matlab function module_dynamic_merge_2018b/Subsystem/statusChecking ==
  data: obj input; caseNum output; ve input; max_dist_gain input; vel_limit input; ttc input; status output
function [caseNum, status] = statusChecking(obj,ve,max_dist_gain,vel_limit,ttc)
    
    id_a = obj.A.ID;
    pa = obj.A.dist ;
    va = obj.A.v;

    id_b = obj.B.ID;
    pb = obj.B.dist ;
    vb = obj.B.v;

    id_c = obj.C.ID ;
    pc = obj.C.dist;
    vc = obj.C.v;

    id_d = obj.D.ID; 
    pd = obj.D.dist;
    vd = obj.D.v;

% in this part, we divide the cases into 4 based on vehicle A and B.
    dtc = ve * max_dist_gain;
    if id_a ~= 0 && id_b ~= 0
        caseNum = 1;
    elseif id_a ~= 0 && id_b == 0
        caseNum = 2;
    elseif id_a == 0 && id_b ~= 0
        caseNum = 3;
    else
        caseNum = 4;
    end

    % check on vehicle A
    if va > ve
        ttc_a = pa / (va - ve);
    else 
        ttc_a = 100;
    end 
            
    % check on vehicle B
    if ve > vb
        ttc_b = pb / (ve - vb);
    else
        ttc_b = 100;
    end
    
    % check on vehicle C
    if ve < vc
        ttc_c = pa / (ve - vc);
    else 
        ttc_c = 100;
    end 
            
    % check on vehicle D
    if vd > va
        ttc_d = pb / (vd - ve);
    else
        ttc_d = 100;
    end
    
    if ttc_c >= ttc && ttc_d >= ttc && (pc >= dtc) && (pd >= dtc)
        adj_flag = 1;
    else
        adj_flag = 0;
    end
    
    switch caseNum
        case 1

            if (ttc_a >= ttc) && (ttc_b >= ttc) ...
                    && (pa >= dtc) && (pb >= dtc) && (ve >= vel_limit)...
                    && (adj_flag == 1)
                
                status = 1;
            else 
                status = 0;
            end
            
        case 2
            
            if (ttc_a >= ttc) && (pa >= dtc) && (ve >= 10)...
                    && (adj_flag == 1) 
                status = 1;
            else 
                status = 0;
            end
            
            
        case 3
           
            if (ttc_b >= ttc) && (pb >= dtc) && (ve >= 10)...
                    && (adj_flag == 1) 
                status = 1;
            else 
                status = 0;
            end
            
            
        otherwise
            if adj_flag == 1
                status = 1;
            else
                status = 0;
            end
  
    end
end

== stateflow chart module_dynamic_merge_2018b/Subsystem/Chart ==
  state initial
    entry:
    Flag = 0;
    isPlanSuc = 0;
  state pre
    entry:
    Flag = 1;
    isPlanSuc = 1;
  state active
    entry:
    Flag = 2;
    isPlanSuc = 2;
  state yield
    entry:
    Flag = 3;
    isPlanSuc = 3;
  (default) -> initial [order 1]
  initial -> pre [order 1] : [trigger == 1  && status ~= 1]
  initial -> active [order 2] : [trigger == 1 && status == 1]
  (default) -> initial [order 2] : [finish == 1]
  active -> initial [order 2] : [finish == 1]
  pre -> active : [status == 1]
  active -> yield [order 1] : [status ~= 1]
  yield -> active : [status == 1]
  data: trigger input double; status input double; finish input double; Flag output double; isPlanSuc output int8
